simulink model "localizeAndControlUsingLidar"  (R2023b)
settings: Solver=VariableStepAuto  StartTime=0.0  StopTime=28.964  RelTol=1e-3
PreLoadFcn:
  | data = load('ReferencePathForward.mat');
  | 
  | load('parkingLotPCMapPoints.mat','ptCloudMapPoints');
  | 
  | startPose = [25.533357  30.0519086033855 180.596809];
  | 
  | helperSLCreateUtilityBus(1);
undefined symbols (not defined in the file or in its folder): centerToRear, curvatures, directions, ptCloudMapPoints, refPoses, velocities
libraries: sim3dautolib x36, drivingvehiclecontroller x2, simulink x2, simulink_extras x2, sim3dphyssensorlib x1, sim3dlib x1, autolibshared x1
(part 2 of 2)

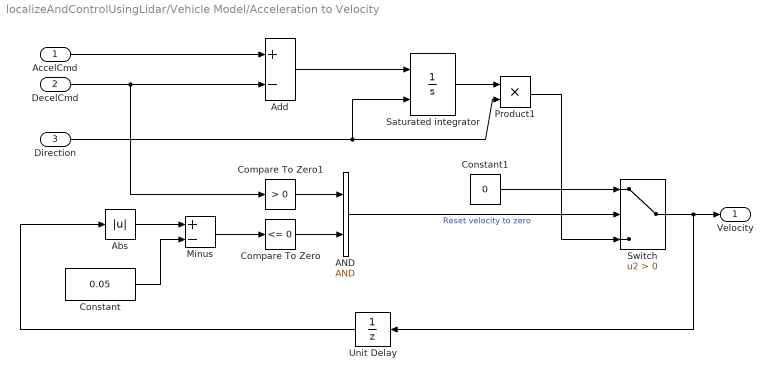
== system localizeAndControlUsingLidar/Vehicle Model/Acceleration to Velocity ==
  AccelCmd : Inport  PortDimensions=[1 1]
  DecelCmd : Inport  Port=2  PortDimensions=[1 1]
  Direction : Inport  Port=3
  AND : Logic  IconShape=distinctive  AllPortsSameDT=off  OutDataTypeStr=boolean
  Abs : Abs  SaturateOnIntegerOverflow=off
  Add : Sum  Inputs=+-
  Compare To Zero : simulink/Logic and Bit Operations/Compare To Zero  relop=<=  OutDataTypeStr=boolean
  Compare To Zero1 : simulink/Logic and Bit Operations/Compare To Zero  relop=>  OutDataTypeStr=boolean
  Constant : Constant  Value=0.05
  Constant1 : Constant  Value=0
  Minus : Sum  Inputs=+-
  Product1 : Product
  Saturated integrator : Integrator  ExternalReset=either  LimitOutput=on  LowerSaturationLimit=0  AbsoluteTolerance=1e-3  ZeroCross=off
  Switch : Switch  Criteria=u2 > Threshold  SaturateOnIntegerOverflow=off  InputSameDT=off
  Unit Delay : UnitDelay  SampleTime=-1  HasFrameUpgradeWarning=on
  Velocity : Outport  VectorParamsAs1DForOutWhenUnconnected=off
  wires:
  Direction/1 -> Product1/2, Saturated integrator/2
  AccelCmd/1 -> Add/1
  Add/1 -> Saturated integrator/1
  DecelCmd/1 -> Compare To Zero1/1, Add/2
  Unit Delay/1 -> Abs/1
  Abs/1 -> Minus/1
  Constant/1 -> Minus/2
  Minus/1 -> Compare To Zero/1
  Compare To Zero/1 -> AND/2
  Compare To Zero1/1 -> AND/1
  AND/1 -> Switch/2  "Reset velocity to zero"
  Switch/1 -> Unit Delay/1, Velocity/1
  Constant1/1 -> Switch/1
  Saturated integrator/1 -> Product1/1
  Product1/1 -> Switch/3

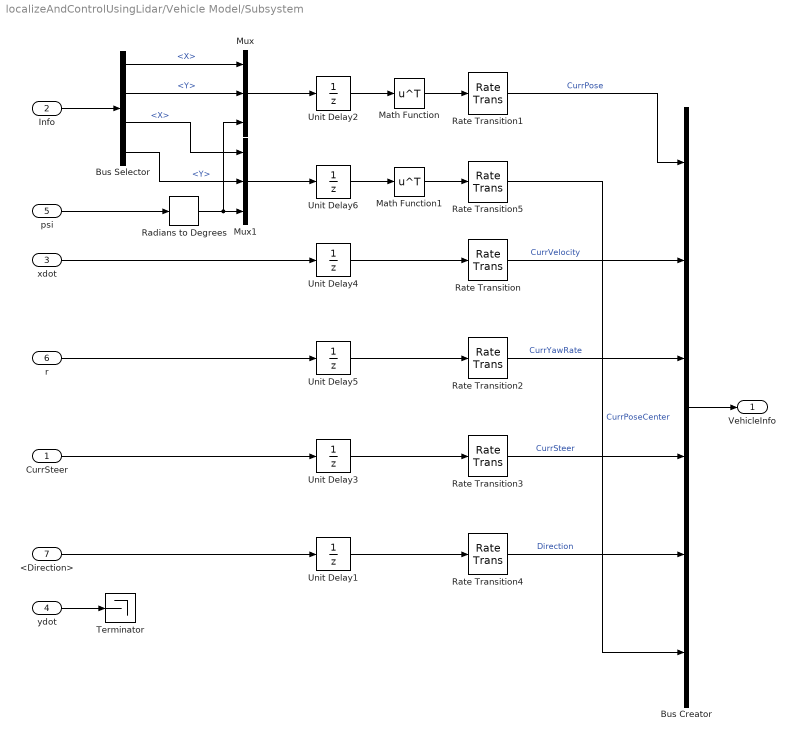
== system localizeAndControlUsingLidar/Vehicle Model/Subsystem ==
  CurrSteer : Inport
  Info : Inport  Port=2
  xdot : Inport  Port=3
  ydot : Inport  Port=4
  psi : Inport  Port=5
  r : Inport  Port=6
  <Direction> : Inport  Port=7
  Bus Creator : BusCreator  Inputs=6  OutDataTypeStr=Bus: vehicleInfoBus  NonVirtualBus=on
  Bus Selector : BusSelector  OutputSignals=InertFrm.RearAxl.Disp.X,InertFrm.RearAxl.Disp.Y,InertFrm.Cg.Disp.X,InertFrm.Cg.Disp.Y
  Math Function : Math  Operator=transpose  SignedPower=on
  Math Function1 : Math  Operator=transpose  SignedPower=on
  Mux : Mux  Inputs=3
  Mux1 : Mux  Inputs=3
  Radians to Degrees : simulink_extras/Transformations/Radians to Degrees
  Rate Transition : RateTransition  OutPortSampleTime=0.05
  Rate Transition1 : RateTransition  InitialCondition=startPose  OutPortSampleTime=0.05
  Rate Transition2 : RateTransition  OutPortSampleTime=0.05
  Rate Transition3 : RateTransition  OutPortSampleTime=0.05
  Rate Transition4 : RateTransition  InitialCondition=1  OutPortSampleTime=0.05
  Rate Transition5 : RateTransition  InitialCondition=[startPose(1)-cosd(startPose(3))*centerToRear,startPose(2)-sind(startPose(3))*centerToRear,startPose(3)]  OutPortSampleTime=0.05
  Terminator : Terminator
  Unit Delay1 : UnitDelay  InitialCondition=1  SampleTime=-1  HasFrameUpgradeWarning=on
  Unit Delay2 : UnitDelay  InitialCondition=startPose  SampleTime=-1  HasFrameUpgradeWarning=on
  Unit Delay3 : UnitDelay  SampleTime=-1  HasFrameUpgradeWarning=on
  Unit Delay4 : UnitDelay  SampleTime=-1  HasFrameUpgradeWarning=on
  Unit Delay5 : UnitDelay  SampleTime=-1  HasFrameUpgradeWarning=on
  Unit Delay6 : UnitDelay  InitialCondition=[startPose(1)-cosd(startPose(3))*centerToRear,startPose(2)-sind(startPose(3))*centerToRear,startPose(3)]  SampleTime=-1  HasFrameUpgradeWarning=on
  VehicleInfo : Outport  VectorParamsAs1DForOutWhenUnconnected=off
  wires:
  Unit Delay1/1 -> Rate Transition4/1
  CurrSteer/1 -> Unit Delay3/1
  Unit Delay5/1 -> Rate Transition2/1
  <Direction>/1 -> Unit Delay1/1
  Unit Delay4/1 -> Rate Transition/1
  Math Function/1 -> Rate Transition1/1
  Rate Transition/1 -> Bus Creator/2  "CurrVelocity"
  Unit Delay3/1 -> Rate Transition3/1
  Rate Transition3/1 -> Bus Creator/4  "CurrSteer"
  Rate Transition1/1 -> Bus Creator/1  "CurrPose"
  Rate Transition2/1 -> Bus Creator/3  "CurrYawRate"
  Rate Transition4/1 -> Bus Creator/5  "Direction"
  Unit Delay2/1 -> Math Function/1
  Info/1 -> Bus Selector/1
  Radians to Degrees/1 -> Mux1/3, Mux/3
  Bus Selector/2 -> Mux/2  "<Y>"
  Bus Selector/1 -> Mux/1  "<X>"
  Mux/1 -> Unit Delay2/1
  xdot/1 -> Unit Delay4/1
  ydot/1 -> Terminator/1
  r/1 -> Unit Delay5/1
  Bus Creator/1 -> VehicleInfo/1
  Bus Selector/4 -> Mux1/2  "<Y>"
  Mux1/1 -> Unit Delay6/1
  Unit Delay6/1 -> Math Function1/1
  Math Function1/1 -> Rate Transition5/1
  Rate Transition5/1 -> Bus Creator/6  "CurrPoseCenter"
  Bus Selector/3 -> Mux1/1  "<X>"
  psi/1 -> Radians to Degrees/1

== matlab function localizeAndControlUsingLidar/MATLAB Function ==
  data: estimatedPose output; xyzPoints input; loc input; or input; mapPoints input
function estimatedPose = localize(xyzPoints,loc,or,mapPoints)
    
    persistent initPose frameCount ndtMap;
    coder.extrinsic("helperLidarLocalizerNDT","pcmapndt","pointCloud","selectSubmap","rigid3d");
    submapSize = [30 30 5];

    if isempty(ndtMap)
        rng(0)
        ptMap = pointCloud(mapPoints);
        ndtMap = pcmapndt(ptMap,1);
    end
    
    if isempty(frameCount)
        frameCount = 0; 
        ndtMap = selectSubmap(ndtMap,loc,submapSize);
        yaw = or(3);
        rot = [cos(yaw), sin(yaw),  0; ...
        -sin(yaw), cos(yaw), 0; ...
        0,         0,    1];
        initPose = rigid3d(rot,loc);
    else
        frameCount = frameCount + 1;
    end
    
    hasNoPoints = all( isnan(xyzPoints), 'all' );
    if hasNoPoints
        estimatedPose = [NaN,NaN,NaN];
        return;
    else
        [ndtMap,x,y,yaw,initPose] = helperLidarLocalizerNDT(xyzPoints,ndtMap,initPose);
        estimatedPose = double([x,y,rad2deg(yaw)]);
    end
end
